simulink model "AGTF30SysDyn_PExPIn"  (R2023b)
settings: Solver=ode4  StartTime=0.0  StopTime=MWS.In.tend  FixedStep=MWS.In.Ts  RelTol=1e-3  EnableMultiTasking=on
model workspace: external: MAT-File (data not in the file)
values from neighbouring files (symbols this model uses):
  MWS = setup_initialize(MWS,startPt,SSsolverSP)    [Setup_Simulation.m]    (also in run_AGTF30e_script.m = Setup_Simulation(inputMethod,MWS.In,filename,Mdl,SSsolverSP))
undefined symbols (not defined in the file or in its folder): DiscIntNeverNeededParam
libraries: simulink x32, Lib_Solve_ModelSource_TMATS x28, Lib_EMTAT x27, Lib_Cntrl_FirstOrderSensor_TMATS x19, Lib_Cntrl_FirstOrderActuator_TMATS x2, Lib_Cntrl_LimitSelect_TMATS x2, Lib_Solve_OuterLoopIntegrator_TMATS x2, Lib_Cntrl_CorrectedSpeed_TMATS x1, Lib_Solve_IterNRSolverJC_TMATS x1, slpidlib x1
(part 8 of 8)

== matlab function AGTF30SysDyn_PExPIn/Actuators/Ring Gear Electric Machine/Rate Limit Enforcement ==
  data: M_preRL input; M_act output; M_old input; Mdot_low input; Mdot_hi input; dt input
function M_act  = fcn(M_preRL,M_old,Mdot_low,Mdot_hi,dt)

M_act = M_preRL;
if (M_preRL < 0 && M_old > 0) || (M_preRL > 0 && M_old < 0)
    M_act = 0;
elseif M_preRL >= 0
    if (M_preRL-M_old)/dt > Mdot_hi
        M_act = M_old + Mdot_hi*dt;
    else
        M_act = M_preRL;
    end
elseif M_preRL < 0
    if (M_preRL-M_old)/dt < Mdot_low
        M_act = M_old + Mdot_low*dt;
    else
        M_act = M_preRL;
    end
end

== matlab function AGTF30SysDyn_PExPIn/Actuators/Carrier Electric Machine/Rate Limit Enforcement ==
  data: M_preRL input; M_act output; M_old input; Mdot_low input; Mdot_hi input; dt input
function M_act  = fcn(M_preRL,M_old,Mdot_low,Mdot_hi,dt)

M_act = M_preRL;
if (M_preRL < 0 && M_old > 0) || (M_preRL > 0 && M_old < 0)
    M_act = 0;
elseif M_preRL >= 0
    if (M_preRL-M_old)/dt > Mdot_hi
        M_act = M_old + Mdot_hi*dt;
    else
        M_act = M_preRL;
    end
elseif M_preRL < 0
    if (M_preRL-M_old)/dt < Mdot_low
        M_act = M_old + Mdot_low*dt;
    else
        M_act = M_preRL;
    end
end

== matlab function AGTF30SysDyn_PExPIn/Actuators/Planet Gear Electric Machine/Rate Limit Enforcement ==
  data: M_preRL input; M_act output; M_old input; Mdot_low input; Mdot_hi input; dt input
function M_act  = fcn(M_preRL,M_old,Mdot_low,Mdot_hi,dt)

M_act = M_preRL;
if (M_preRL < 0 && M_old > 0) || (M_preRL > 0 && M_old < 0)
    M_act = 0;
elseif M_preRL >= 0
    if (M_preRL-M_old)/dt > Mdot_hi
        M_act = M_old + Mdot_hi*dt;
    else
        M_act = M_preRL;
    end
elseif M_preRL < 0
    if (M_preRL-M_old)/dt < Mdot_low
        M_act = M_old + Mdot_low*dt;
    else
        M_act = M_preRL;
    end
end
